simulink model "adpmodel"  (R2016b)
settings: Solver=VariableStepAuto  StartTime=0.0  StopTime=10.0  RelTol=1e-3
values from neighbouring files (symbols this model uses):
  A = [0 1; -0.1 0.1]    [main.m]
  B = [0;1]    [main.m]
  C = eye(2)    [main.m]
  D = [0;0]    [main.m]
  Q = eye(2)    [main.m]
  R = 1    [main.m]
  x0 = [0;0]    [main.m]
settings Model: Creator=Yuri  LastModifiedBy=Yuri

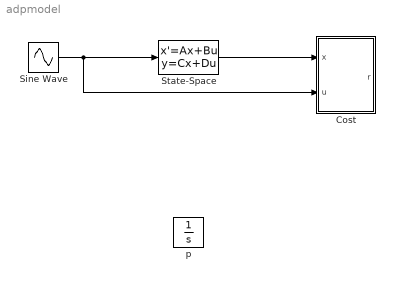
== system adpmodel ==
  "Cost " : Subsystem
  Sine Wave : Sin  SampleTime=0
  State-Space : StateSpace  A=A  B=B  C=C  D=D  X0=x0
  p : Integrator
  wires:
  State-Space/1 -> "Cost "/1(x)
  Sine Wave/1 -> "Cost "/2(u), State-Space/1

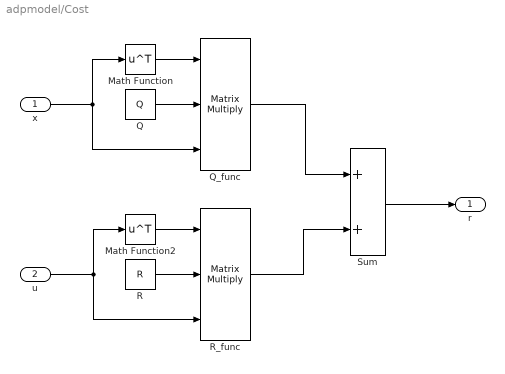
== system adpmodel/Cost  ==
  x : Inport
  u : Inport  Port=2
  Math Function : Math  Operator=transpose  SaturateOnIntegerOverflow=on
  Math Function2 : Math  Operator=transpose  SaturateOnIntegerOverflow=on
  Q : Constant  Value=Q
  Q_func : Product  Inputs=3  Multiplication=Matrix(*)
  R : Constant  Value=R
  R_func : Product  Inputs=3  Multiplication=Matrix(*)
  Sum : Sum
  r : Outport
  wires:
  Q/1 -> Q_func/2
  R/1 -> R_func/2
  Sum/1 -> r/1
  Q_func/1 -> Sum/1
  R_func/1 -> Sum/2
  x/1 -> Q_func/3, Math Function/1
  u/1 -> R_func/3, Math Function2/1
  Math Function/1 -> Q_func/1
  Math Function2/1 -> R_func/1
